simulink model "Trajectory_tracking"  (R2021b)
settings: Solver=VariableStepAuto  StartTime=0.0  StopTime=10.0  RelTol=1e-3
libraries: matrix_library x1
settings Model: Creator=hp  LastModifiedBy=hp

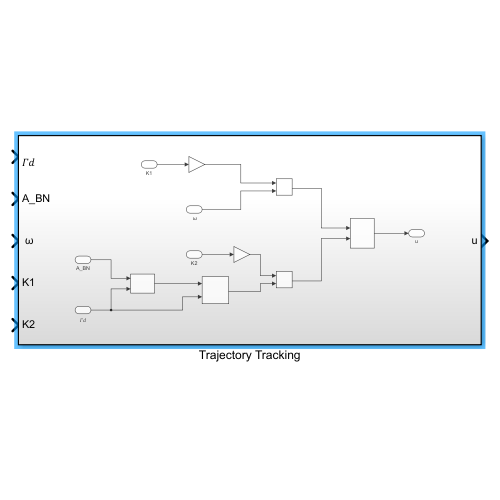
[thumbnail: Simulink's stored preview of the top-level diagram]
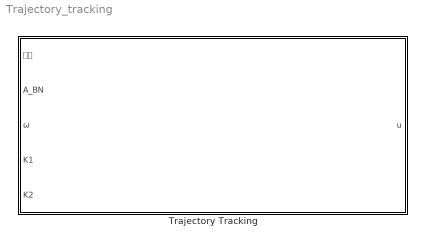
== system Trajectory_tracking ==
  Trajectory Tracking : Subsystem

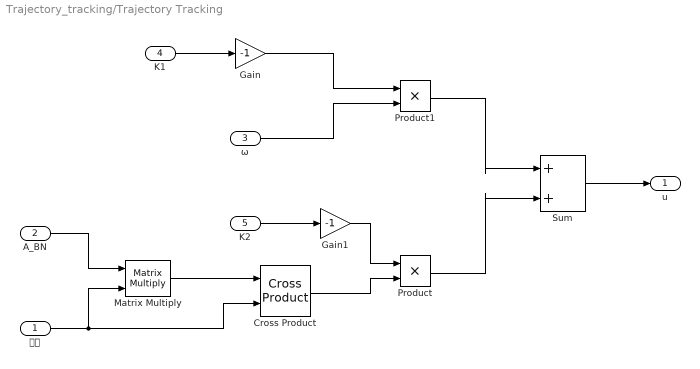
== system Trajectory_tracking/Trajectory Tracking ==
  𝛤𝑑 : Inport
  A_BN : Inport  Port=2
  " ω" : Inport  Port=3
  K1 : Inport  Port=4
  K2 : Inport  Port=5
  Cross Product : matrix_library/Cross Product
      settings: SourceProductBaseCode=SL
  Gain : Gain  Gain=-1
  Gain1 : Gain  Gain=-1
  Matrix Multiply : Product  Multiplication=Matrix(*)
  Product : Product
  Product1 : Product
  Sum : Sum  Inputs=|+|+|
  u : Outport
  wires:
  𝛤𝑑/1 -> Cross Product/2, Matrix Multiply/2
  A_BN/1 -> Matrix Multiply/1
  K1/1 -> Gain/1
  K2/1 -> Gain1/1
  Matrix Multiply/1 -> Cross Product/1
  Cross Product/1 -> Product/2
  Gain1/1 -> Product/1
  Gain/1 -> Product1/1
  " ω"/1 -> Product1/2
  Product1/1 -> Sum/1
  Product/1 -> Sum/2
  Sum/1 -> u/1
